simulink model "Problem2"  (R2020b)
settings: Solver=VariableStepAuto  StartTime=0.0  StopTime=50  RelTol=1e-3
settings Model: Creator=ARPITA  LastModifiedBy=ARPITA

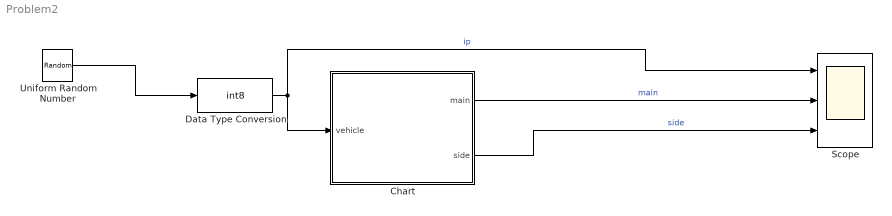
== system Problem2 ==
  Chart : Stateflow chart  TreatAsAtomicUnit=on
  Data Type Conversion : DataTypeConversion  OutDataTypeStr=int8
  Scope : Scope  NumInputPorts=3
  Uniform Random Number : UniformRandomNumber  Minimum=0  Maximum=5  Seed=30  SampleTime=1
  wires:
  Uniform Random Number/1 -> Data Type Conversion/1
  Data Type Conversion/1 -> Scope/1, Chart/1(vehicle)  "ip"
  Chart/2(side) -> Scope/3  "side"
  Chart/1(main) -> Scope/2  "main"

== stateflow chart Problem2/Chart ==
  settings: stateMachineType=MOORE_MACHINE
  state FirstState
    main = GREEN;
    side = RED;
  state SecondState
    main = YELLOW;
    side = RED;
  state ThirdState
    main = RED;
    side = RED;
  state SixthState
    main = RED;
    side = RED;
  state FifthState
    main = RED;
    side = YELLOW;
  state FourthState
    main = RED;
    side = GREEN;
  (default) -> FirstState
  FirstState -> SecondState : [vehicle==1 || after(25,tick)]
  SecondState -> ThirdState : after(4,tick)
  SixthState -> FirstState : after(1,tick)
  ThirdState -> FourthState : after(1,tick)
  FifthState -> SixthState : after(4,tick)
  FourthState -> FifthState : [vehicle==0 && after(25,tick)]
  data: vehicle input; GREEN constant double =3; YELLOW constant double =2; RED constant double =1; main output; side output
